simulink model "PositionLoop_code_202407156_v18b"  (R2018b)
settings: Solver=ode4  StartTime=0.0  StopTime=100  FixedStep=0.00025  RelTol=1e-3
libraries: simulink x2, dspstat3 x1, discretizing x1
settings Model: Creator=randolf  LastModifiedBy=randolf
settings DataIOCC: ReturnWorkspaceOutputs=on
settings OptimizationCC: DefaultParameterBehavior=Inlined  UseDivisionForNetSlopeComputation=on  UseFloatMulNetSlope=on  InlineInvariantSignals=on  PassReuseOutputArgsAs=Individual arguments  ZeroExternalMemoryAtStartup=off  ZeroInternalMemoryAtStartup=off  NoFixptDivByZeroProtection=on  EfficientFloat2IntCast=on  LifeSpan=1  OptimizeBlockOrder=speed  DifferentSizesBufferReuse=on
settings DebuggingCC: ParameterTunabilityLossMsg=error  UnconnectedInputMsg=none  UnconnectedOutputMsg=none  UnconnectedLineMsg=none  SFMachineParentedDataDiag=error
settings HardwareCC: ProdBitPerPointer=32  ProdBitPerSizeT=32  ProdBitPerPtrDiffT=32  ProdLargestAtomicInteger=Long  ProdLargestAtomicFloat=Double  ProdWordSize=32  ProdLongLongMode=on  ProdHWDeviceType=ARM Compatible->ARM Cortex-M
settings SFSimCC: MATLABDynamicMemAlloc=off
settings RTWCC: SystemTargetFile=ert.tlc  TemplateMakefile=ert_default_tmf
settings CodeAppCC: ForceParamTrailComments=on  IgnoreCustomStorageClasses=off  OperatorAnnotations=on  SimulinkDataObjDesc=on  SFDataObjDesc=on  CustomSymbolStrGlobalVar=rt$N$M  CustomSymbolStrType=$N$M  CustomSymbolStrFcn=$N$M$F  CustomSymbolStrFcnArg=$R_rt$I$N$M  CustomSymbolStrMacro=$N$M  InsertBlockDesc=on
settings ERTTargetCC: TargetLangStandard=C99 (ISO)  GenerateSampleERTMain=on  IncludeMdlTerminateFcn=off  CombineSignalStateStructs=on  CodeInterfacePackaging=Reusable function  SupportComplex=off  SupportContinuousTime=on  SupportNonInlinedSFcns=on  InlinedParameterPlacement=NonHierarchical  ERTCustomFileTemplate=example_file_process.tlc  ERTFilePackagingFormat=CompactWithDataFile

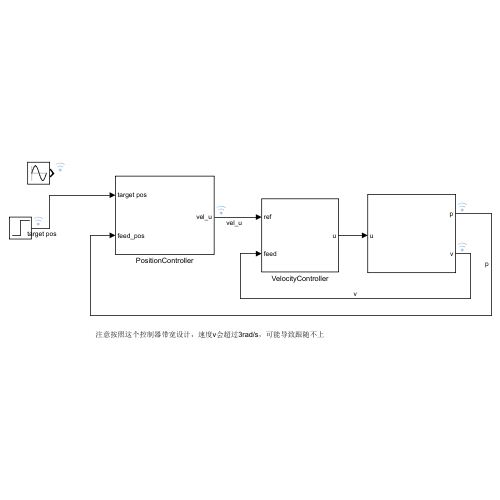
[thumbnail: Simulink's stored preview of the top-level diagram]
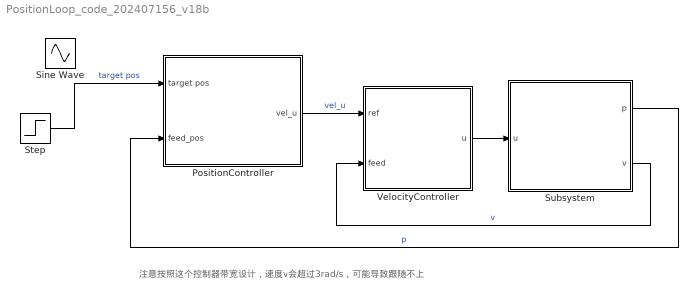
== system PositionLoop_code_202407156_v18b ==
  note: 注意按照这个控制器带宽设计，速度v会超过3rad/s，可能导致跟随不上
  PositionController : Subsystem
  Sine Wave : Sin  Frequency=2  SampleTime=0
  Step : Step  SampleTime=0
  Subsystem : Subsystem
  VelocityController : Subsystem
  wires:
  VelocityController/1(u) -> Subsystem/1(u)
  Subsystem/2(v) -> VelocityController/2(feed)  "v"
  Step/1 -> PositionController/1(target pos)  "target pos"
  Subsystem/1(p) -> PositionController/2(feed_pos)  "p"
  PositionController/1(vel_u) -> VelocityController/1(ref)  "vel_u"

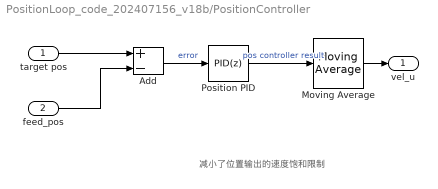
== system PositionLoop_code_202407156_v18b/PositionController ==
  note: 减小了位置输出的速度饱和限制
  target pos : Inport  PortDimensions=1
  feed_pos : Inport  Port=2  PortDimensions=1
  Add : Sum  Inputs=+-
  Moving Average : dspstat3/Moving Average  Method=Exponential weighting  ForgettingFactorPort=off  SpecifyWindowLength=on  WindowLength=4  ForgettingFactor=0.99  SimulateUsing=Code generation
  Position PID : simulink/Continuous/PID Controller  Controller=PID  Form=Parallel  TimeDomain=Discrete-time  SampleTime=0.00050000000000000001  IntegratorMethod=Forward Euler  ControllerParametersSource=internal  P=36.642474191182998  I=260.653872931600006  D=0.381884424337911  N=1796.585349822470789  UseFilter=on  TunerSelectOption=Transfer Function Based (PID Tuner App)  InitialConditionSource=internal  InitialConditionForIntegrator=0  InitialConditionForFilter=0  DifferentiatorICPrevScaledInput=0  ExternalReset=none  TrackingMode=off  Kt=1  LimitOutput=on  UpperSaturationLimit=2  LowerSaturationLimit=-2  LinearizeAsGain=on  AntiWindupMode=clamping  Kb=1  POutMin=[]  POutMax=[]  IOutMin=[]  IOutMax=[]  DOutMin=[]  DOutMax=[]  NOutMin=[]  NOutMax=[]  SumOutMin=[]  SumOutMax=[]  SaturationOutMin=[]  SaturationOutMax=[]  PParamMin=[]  PParamMax=[]  IParamMin=[]  IParamMax=[]  DParamMin=[]  DParamMax=[]  NParamMin=[]  NParamMax=[]  KbParamMin=[]  KbParamMax=[]  KtParamMin=[]  KtParamMax=[]  KbOutMin=[]  KbOutMax=[]  KtOutMin=[]  KtOutMax=[]  IntegratorOutMin=[]  IntegratorOutMax=[]  FilterOutMin=[]  FilterOutMax=[]  SumI1OutMin=[]  SumI1OutMax=[]  SumI2OutMin=[]  SumI2OutMax=[]  SumI3OutMin=[]  SumI3OutMax=[]  SumI4OutMin=[]  SumI4OutMax=[]  SumDOutMin=[]  SumDOutMax=[]  DifferentiatorOutMin=[]  DifferentiatorOutMax=[]  FilterDiffOutCoefMin=[]  FilterDiffOutCoefMax=[]  ReciprocalOutMin=[]  ReciprocalOutMax=[]  SumDenOutMin=[]  SumDenOutMax=[]  SumNumOutMin=[]  SumNumOutMax=[]  DivideOutMin=[]  DivideOutMax=[]  IntegratorContinuousStateAttributes=''  IntegratorStateMustResolveToSignalObject=off  IntegratorRTWStateStorageClass=Auto  FilterContinuousStateAttributes=''  FilterStateMustResolveToSignalObject=off  FilterRTWStateStorageClass=Auto  ParallelPVariant=InternalParameters  IdealPVariant=Disabled  IVariant=InternalParameters  DVariant=InternalParameters  IntegratorVariant=Discrete  SatVariant=Enabled  AWVariant=DiscClampingParallel  PCopyVariant=Disabled  TRVariant=Disabled  FdbkBlocksVariant=Forward  IdealPFdbkVariant=Disabled  SatFdbkVariant=Disabled  DerivativeFilterVariant=ForwardEulerFilter  NVariant=InternalParameters  NCopyVariant=Disabled  FilterICVariant=InternalICsFilter  IntegratorICVariant=InternalICs  ExternalResetVariant=Disabled  TRSumVariant=Passthrough  SumFdbkVariant=Disabled  SumVariant=Sum_PID
  vel_u : Outport  PortDimensions=1
  wires:
  target pos/1 -> Add/1
  Add/1 -> Position PID/1  "error"
  Position PID/1 -> Moving Average/1  "pos controller result"
  feed_pos/1 -> Add/2
  Moving Average/1 -> vel_u/1

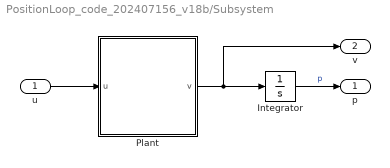
== system PositionLoop_code_202407156_v18b/Subsystem ==
  u : Inport
  Integrator : Integrator
  Plant : Subsystem
  p : Outport
  v : Outport  Port=2
  wires:
  Plant/1(v) -> v/1, Integrator/1
  Integrator/1 -> p/1  "p"
  u/1 -> Plant/1(u)

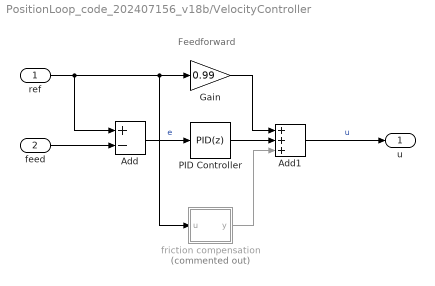
== system PositionLoop_code_202407156_v18b/VelocityController ==
  note: Feedforward
  ref : Inport
  feed : Inport  Port=2
  Add : Sum  Inputs=+-
  Add1 : Sum  Inputs=+++
  Gain : Gain  Gain=0.99
  PID Controller : simulink/Continuous/PID Controller  Controller=PID  Form=Parallel  TimeDomain=Discrete-time  SampleTime=0.00025  IntegratorMethod=Forward Euler  ControllerParametersSource=internal  P=992.697353800287  I=9306.57767463189  D=1.45672350385708  N=98.7705129393937  UseFilter=on  TunerSelectOption=Transfer Function Based (PID Tuner App)  InitialConditionSource=internal  InitialConditionForIntegrator=0  InitialConditionForFilter=0  DifferentiatorICPrevScaledInput=0  ExternalReset=none  TrackingMode=off  Kt=1  LimitOutput=on  UpperSaturationLimit=1000  LowerSaturationLimit=-1000  LinearizeAsGain=on  AntiWindupMode=clamping  Kb=1  POutMin=[]  POutMax=[]  IOutMin=[]  IOutMax=[]  DOutMin=[]  DOutMax=[]  NOutMin=[]  NOutMax=[]  SumOutMin=[]  SumOutMax=[]  SaturationOutMin=[]  SaturationOutMax=[]  PParamMin=[]  PParamMax=[]  IParamMin=[]  IParamMax=[]  DParamMin=[]  DParamMax=[]  NParamMin=[]  NParamMax=[]  KbParamMin=[]  KbParamMax=[]  KtParamMin=[]  KtParamMax=[]  KbOutMin=[]  KbOutMax=[]  KtOutMin=[]  KtOutMax=[]  IntegratorOutMin=[]  IntegratorOutMax=[]  FilterOutMin=[]  FilterOutMax=[]  SumI1OutMin=[]  SumI1OutMax=[]  SumI2OutMin=[]  SumI2OutMax=[]  SumI3OutMin=[]  SumI3OutMax=[]  SumI4OutMin=[]  SumI4OutMax=[]  SumDOutMin=[]  SumDOutMax=[]  DifferentiatorOutMin=[]  DifferentiatorOutMax=[]  FilterDiffOutCoefMin=[]  FilterDiffOutCoefMax=[]  ReciprocalOutMin=[]  ReciprocalOutMax=[]  SumDenOutMin=[]  SumDenOutMax=[]  SumNumOutMin=[]  SumNumOutMax=[]  DivideOutMin=[]  DivideOutMax=[]  IntegratorContinuousStateAttributes=''  IntegratorStateMustResolveToSignalObject=off  IntegratorRTWStateStorageClass=Auto  FilterContinuousStateAttributes=''  FilterStateMustResolveToSignalObject=off  FilterRTWStateStorageClass=Auto  ParallelPVariant=InternalParameters  IdealPVariant=Disabled  IVariant=InternalParameters  DVariant=InternalParameters  IntegratorVariant=Discrete  SatVariant=Enabled  AWVariant=DiscClampingParallel  PCopyVariant=Disabled  TRVariant=Disabled  FdbkBlocksVariant=Forward  IdealPFdbkVariant=Disabled  SatFdbkVariant=Disabled  DerivativeFilterVariant=ForwardEulerFilter  NVariant=InternalParameters  NCopyVariant=Disabled  FilterICVariant=InternalICsFilter  IntegratorICVariant=InternalICs  ExternalResetVariant=Disabled  TRSumVariant=Passthrough  SumFdbkVariant=Disabled  SumVariant=Sum_PID
  friction compensation : MATLAB Function  Commented=on  TreatAsAtomicUnit=on
  u : Outport
  wires:
  Add/1 -> PID Controller/1  "e"
  friction compensation/1(y) -> Add1/3
  Add1/1 -> u/1  "u"
  Gain/1 -> Add1/1
  feed/1 -> Add/2
  ref/1 -> Add/1, friction compensation/1(u), Gain/1
  PID Controller/1 -> Add1/2

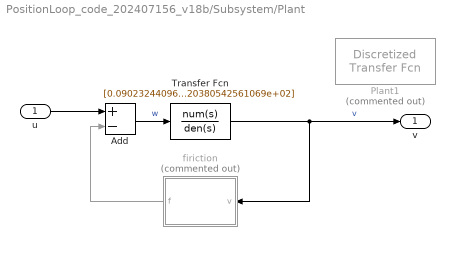
== system PositionLoop_code_202407156_v18b/Subsystem/Plant ==
  u : Inport
  Add : Sum  Inputs=+-
  Plant1 : discretizing/Discretized Transfer Fcn  Commented=on  Numerator=[0.090232440960097,3.051715207136733,19.382986592459790]  Denominator=[1,20.527749511328590,2.672042521178649e+02,7.720380542561069e+02]  AbsTol=auto  SampleTime=0.0002  method=zoh  Wc=1
      settings: SourceProductBaseCode=SL
  Transfer Fcn : TransferFcn  Numerator=[0.090232440960097,3.051715207136733,19.382986592459790]  Denominator=[1,20.527749511328590,2.672042521178649e+02,7.720380542561069e+02]
  firiction : MATLAB Function  Commented=on  TreatAsAtomicUnit=on
  v : Outport
  wires:
  Add/1 -> Transfer Fcn/1  "w"
  u/1 -> Add/1
  Transfer Fcn/1 -> firiction/1(v), v/1  "v"
  firiction/1(f) -> Add/2

== matlab function PositionLoop_code_202407156_v18b/VelocityController/friction compensation ==
  data: u input; y output
function y = fcn(u)
    v_band = 0.005;
    if (abs(u) > v_band)
        if (u > 0)
            y = 154;
        else
            y = -154;
        end
    else
        y = 154 * tanh(u/v_band)/tanh(1);
    end

end

== matlab function PositionLoop_code_202407156_v18b/Subsystem/Plant/firiction ==
  data: v input; f output
function f = fcn(v)
    if (v>0)
        f = 153;
    else
        f = -154;
    end
end
